simulink model "Fuzzy_and_EKF_STOCAZZO"  (R2021b)
settings: Solver=ode4  StartTime=0.0  StopTime=10.0  FixedStep=1e-2  RelTol=1e-3
values from neighbouring files (symbols this model uses):
  n = length(out.tout)    [Plot_dati.m]
undefined symbols (not defined in the file or in its folder): measure
libraries: fuzblock x1
settings Model: Creator=francescoiotti  LastModifiedBy=pierg
settings ModelReferenceCC: ModelReferenceMinAlgLoopOccurrences=on

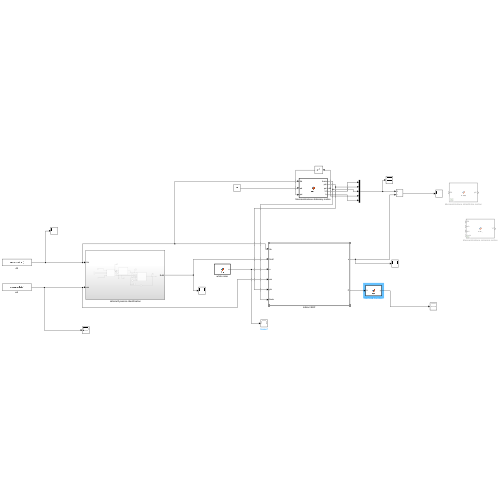
[thumbnail: Simulink's stored preview of the top-level diagram]
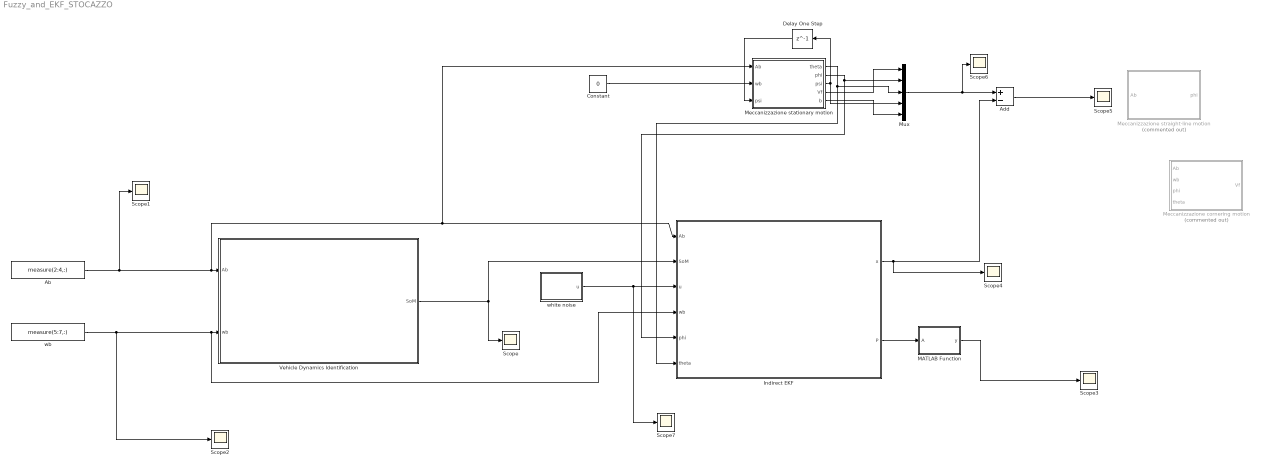
== system Fuzzy_and_EKF_STOCAZZO ==
  Ab : Constant  Value=measure(2:4,:)
  Add : Sum  Inputs=+-
  Constant : Constant  Value=0
  Delay One Step : Delay  DelayLength=1
  Indirect EKF : Subsystem
  MATLAB Function : MATLAB Function  TreatAsAtomicUnit=on
  Meccanizzazione cornering motion : MATLAB Function  Commented=on  TreatAsAtomicUnit=on
  Meccanizzazione stationary motion : MATLAB Function  TreatAsAtomicUnit=on
  Meccanizzazione straight-line motion : MATLAB Function  Commented=on  TreatAsAtomicUnit=on
  Mux : Mux  Inputs=5
  Scope{,1..7} (8 alike) : Scope
  Vehicle Dynamics Identification : Subsystem
  wb : Constant  Value=measure(5:7,:)
  white noise : MATLAB Function  TreatAsAtomicUnit=on
  wires:
  Vehicle Dynamics Identification/1(SoM) -> Indirect EKF/2(SoM), Scope/1
  Ab/1 -> Indirect EKF/1(Ab), Meccanizzazione stationary motion/1(Ab), Vehicle Dynamics Identification/1(Ab), Scope1/1
  wb/1 -> Indirect EKF/4(wb), Vehicle Dynamics Identification/2(wb), Scope2/1
  Indirect EKF/1(x) -> Scope4/1, Add/2
  Indirect EKF/2(P) -> MATLAB Function/1(A)
  Meccanizzazione stationary motion/1(theta) -> Indirect EKF/6(theta), Mux/3
  Meccanizzazione stationary motion/2(phi) -> Indirect EKF/5(phi), Mux/2
  Meccanizzazione stationary motion/3(psi) -> Mux/4, Delay One Step/1
  Delay One Step/1 -> Meccanizzazione stationary motion/3("psi ")
  Meccanizzazione stationary motion/4(Vf) -> Mux/1
  Meccanizzazione stationary motion/5(b) -> Mux/5
  Mux/1 -> Scope6/1, Add/1
  Add/1 -> Scope5/1
  white noise/1(u) -> Indirect EKF/3(u), Scope7/1
  Constant/1 -> Meccanizzazione stationary motion/2(wb)
  MATLAB Function/1(y) -> Scope3/1

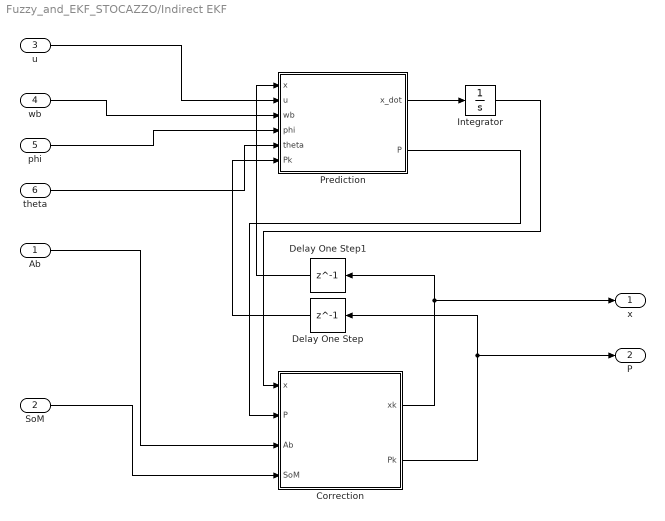
== system Fuzzy_and_EKF_STOCAZZO/Indirect EKF ==
  Ab : Inport
  SoM : Inport  Port=2
  u : Inport  Port=3
  wb : Inport  Port=4
  phi : Inport  Port=5
  theta : Inport  Port=6
  Correction : MATLAB Function  TreatAsAtomicUnit=on
  Delay One Step : Delay  DelayLength=1
  Delay One Step1 : Delay  DelayLength=1
  Integrator : Integrator  InitialCondition=[0 0 0 0 0]'
  Prediction : MATLAB Function  InitFcn=Pk = eye(5)  TreatAsAtomicUnit=on
  x : Outport
  P : Outport  Port=2
  wires:
  Prediction/1(x_dot) -> Integrator/1
  Integrator/1 -> Correction/1(x)
  Ab/1 -> Correction/3(Ab)
  SoM/1 -> Correction/4(SoM)
  Correction/1(xk) -> Delay One Step1/1, x/1
  Correction/2(Pk) -> Delay One Step/1, P/1
  u/1 -> Prediction/2(u)
  Prediction/2(P) -> Correction/2(P)
  wb/1 -> Prediction/3(wb)
  phi/1 -> Prediction/4(phi)
  theta/1 -> Prediction/5(theta)
  Delay One Step/1 -> Prediction/6(Pk)
  Delay One Step1/1 -> Prediction/1(x)

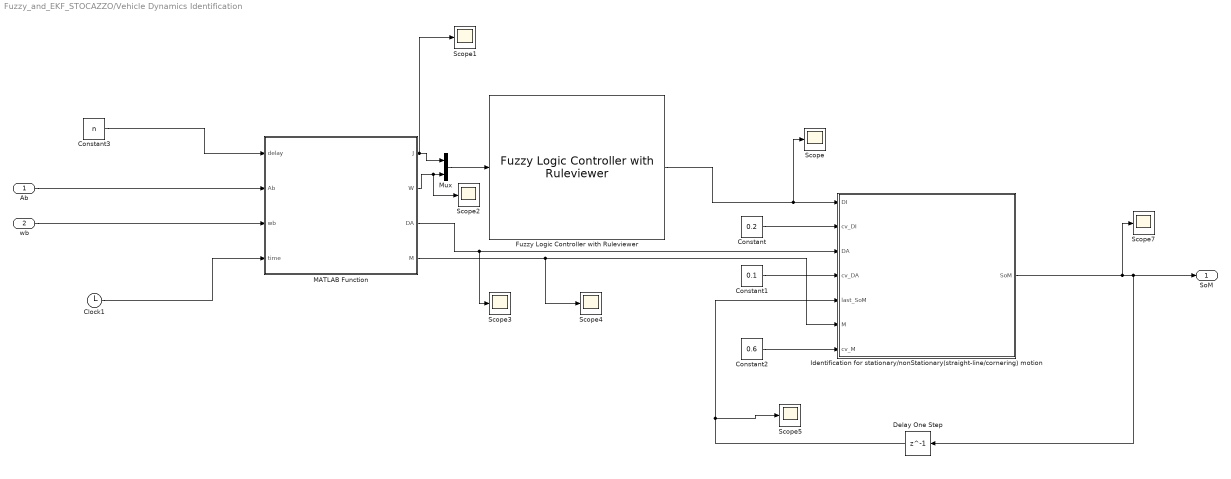
== system Fuzzy_and_EKF_STOCAZZO/Vehicle Dynamics Identification ==
  Ab : Inport
  wb : Inport  Port=2
  Clock1 : Clock
  Constant : Constant  Value=0.2
  Constant1 : Constant  Value=0.1
  Constant2 : Constant  Value=0.6
  Constant3 : Constant  Value=n
  Delay One Step : Delay  DelayLength=1  InitialCondition=1
  Fuzzy Logic Controller with Ruleviewer : fuzblock/Fuzzy Logic  Controller  with Ruleviewer  fismatrix=pippo  Ts=5
  Identification for stationary/nonStationary(straight-line/cornering) motion : MATLAB Function  TreatAsAtomicUnit=on
  MATLAB Function : MATLAB Function  TreatAsAtomicUnit=on
  Mux : Mux  Inputs=2
  Scope{,1..5,7} (7 alike) : Scope
  SoM : Outport
  wires:
  Constant1/1 -> Identification for stationary/nonStationary(straight-line/cornering) motion/4(cv_DA)
  MATLAB Function/3(DA) -> Scope3/1, Identification for stationary/nonStationary(straight-line/cornering) motion/3(DA)
  MATLAB Function/1(J) -> Scope1/1, Mux/1
  Fuzzy Logic Controller with Ruleviewer/1 -> Scope/1, Identification for stationary/nonStationary(straight-line/cornering) motion/1(DI)
  MATLAB Function/4(M) -> Scope4/1, Identification for stationary/nonStationary(straight-line/cornering) motion/6(M)
  Identification for stationary/nonStationary(straight-line/cornering) motion/1(SoM) -> Scope7/1, SoM/1, Delay One Step/1
  Constant2/1 -> Identification for stationary/nonStationary(straight-line/cornering) motion/7(cv_M)
  Constant/1 -> Identification for stationary/nonStationary(straight-line/cornering) motion/2(cv_DI)
  MATLAB Function/2(W) -> Scope2/1, Mux/2
  Mux/1 -> Fuzzy Logic Controller with Ruleviewer/1
  Clock1/1 -> MATLAB Function/4(time)
  wb/1 -> MATLAB Function/3(wb)
  Ab/1 -> MATLAB Function/2(Ab)
  Constant3/1 -> MATLAB Function/1(delay)
  Delay One Step/1 -> Scope5/1, Identification for stationary/nonStationary(straight-line/cornering) motion/5(last_SoM)

== matlab function Fuzzy_and_EKF_STOCAZZO/MATLAB Function ==
  data: A input; y output
function y = fcn(A)
y = norm(A);

== matlab function Fuzzy_and_EKF_STOCAZZO/Meccanizzazione straight-line motion ==
  data: Ab input; phi output
function phi  = mecc(Ab)
% Estraggo le componenti di accelerazione
Abx = Ab(1);
Aby = Ab(2);

% Estraggo le componenti di velocità angolare
% wbx = wb(1);
% wby = wb(2);
% wbz = wb(3);

% Costante
g = 9.81;

% Meccanizzazione
phi = asin(-Aby / sqrt(g^2 - Abx^2));

== matlab function Fuzzy_and_EKF_STOCAZZO/Meccanizzazione stationary motion ==
  data: Ab input; theta output; wb input; psi input; phi output; psi output; Vf output; b output
function [theta, phi, psi, Vf, b] = mecc(Ab, wb, psi)
% Estraggo le componenti di accelerazione
Abx = Ab(1);
Aby = Ab(2);

% Estraggo le componenti di velocità angolare
% wbx = wb(1);
% wby = wb(2);
% wbz = wb(3);

% Costante
g = 9.81;

% Meccanizzazione
theta = asin(Abx/g);
phi = asin(-Aby / sqrt(g^2 - Abx^2));
psi = psi;
Vf = 0;
b = wb;

== matlab function Fuzzy_and_EKF_STOCAZZO/Vehicle Dynamics Identification/Identification for stationary//nonStationary(straight-line//cornering) motion ==
  data: DI input; cv_DI input; DA input; cv_DA input; last_SoM input; M input; SoM output; cv_M input
function SoM = type_of_motion_decision_loop(DI, cv_DI, DA, cv_DA, last_SoM, M, cv_M)

    %% Identification for stationary/nonStationary(straight-line/cornering) motion
    % SoM : state of motion for landend vehicle
    % last_SoM: previous state of motion for landend vehicle
    % 0 := Stationary
    % 1 := straight-line motion
    % 2 := cornering motion
    % notStationary: if 1 the vehicle is not stationary

    notStationary = 1;
    SoM = 0;

    if last_SoM == 0 && DA > cv_DA      
        notStationary = 1;
    elseif	last_SoM && DA < cv_DA && DI < cv_DI
        SoM = 0;
        notStationary = 0;
    else 
        SoM = last_SoM;
        notStationary = 0;
    end
    
    %Run this only if notStactionary
    if notStationary && M > cv_M
        SoM = 2;
    elseif	notStationary && M < cv_M
        SoM = 1;
    elseif notStationary 
        SoM = last_SoM;
    end

    notStationary

== matlab function Fuzzy_and_EKF_STOCAZZO/Vehicle Dynamics Identification/MATLAB Function ==
  data: delay input; Ab input; J output; wb input; time input; W output; DA output; M output
function [J, W, DA, M] = functional_computation(delay, Ab, wb, time)
% Trasformo i tempi in passi
n = int64(delay/1e-2);
t = int64(time/1e-2);
p = int64(1/30/1e-2);
m = n;
% Inizializzo i funzionali
J = 0;
W = 0;
DA = 0;
Mwbz = 0;

% Calcolo J
for i=t-n:t
%   Controllo nel caso in cui t < n ed escludo i termini con indici
%   negativi
    if i > 1
        J = J + abs( norm(Ab(:,i)) - norm(Ab(:,i-1)) );
    end
end

% Calcolo W
for i=t-n:t
%   Controllo nel caso in cui t < n ed escludo i termini con indici
%   negativi
    if i > 1
        W = W + abs( sqrt(wb(1,i)^2 + wb(2,i)^2) ) / double(n);
    end
end


% Calcolo DA
for i=t-p:t
%   Controllo nel caso in cui t < n ed escludo i termini con indici
%   negativi
    if i > 1 && t-p > 0
        DA = DA + abs( Ab(1,i) - Ab(1,t-p) );
    end
end


% Calcolo M
for i=t-m:t
%   Controllo nel caso in cui t < n ed escludo i termini con indici
%   negativi
    if i > 1
        Mwbz = Mwbz + wb(3,i);
    end
end
M = Mwbz / m;

== matlab function Fuzzy_and_EKF_STOCAZZO/Meccanizzazione cornering motion ==
  data: Ab input; wb input; phi input; Vf output; theta input
function Vf  = mecc(Ab, wb, phi, theta)
% Estraggo le componenti di accelerazione
%Abx = Ab(1);
Aby = Ab(2);

% Estraggo le componenti di velocità angolare
% wbx = wb(1);
% wby = wb(2);
wbz = wb(3);

% Costante
g = 9.81;

% Meccanizzazione
Vf = (Aby + g*sin(phi)*cos(theta)) / wbz;

== matlab function Fuzzy_and_EKF_STOCAZZO/Indirect EKF/Prediction ==
  data: x_dot output; x input; u input; wb input; phi input; theta input; Pk input; P output
function [x_dot, P] = prediction(x, u, wb, phi, theta, Pk)

% Estraggo le componenti di velocità angolare
wbx = wb(1);
wby = wb(2);
wbz = wb(3);

% Costante
g = 9.81;

% Definisco gli elementi della matrice F
f13 = -g*cos(theta);
f22 = cos(phi)*tan(theta)*wby - sin(phi)*tan(theta)*wbz;
f23 = sin(phi)*wby/cos(theta)^2 + cos(phi)*wbz/cos(theta)^2;
f32 = -sin(phi)*wby - cos(phi)*wbz;
f42 = cos(phi)*wby/cos(theta) - sin(phi)*wbz/cos(theta);
f43 = sin(phi)*tan(theta)*wby/cos(theta) + cos(phi)*tan(theta)*wbz/cos(theta);

F = [0  0  f13  0  1;
     0 f22 f23  0  0;
     0 f32  0   0  0;
     0 f42 f43  0  0;
     0  0   0   0  0;];

% Definisco gli elementi della matrice G
g23 = sin(phi)*tan(theta);
g24 = cos(phi)*tan(theta);
g33 = cos(phi);
g34 = -sin(phi);
g43 = sin(phi)/cos(theta);
g44 = cos(phi)/cos(theta);

G = [1  0  0   0  0;
     0  1 g23 g24 0;
     0  0 g33 g34 0;
     0  0 g43 g44 0;
     0  0  0   0  1;];

% Formula di predizione dello stato
x_dot = F*x + G*u;


% Definisco la matrice di covarianza del rumore di processo Q
qAbx = 0.001; % densità spettrale
qwbx = 0.1;
qwby = 0.1;
qwbz = 0.1;
qb = 0;
Q = diag([qAbx, qwbx, qwby, qwbz, qb]);

% Formula di predizione della covarianza
P = F*Pk*F' + Q;

== matlab function Fuzzy_and_EKF_STOCAZZO/Indirect EKF/Correction ==
  data: x input; xk output; P input; Ab input; Pk output; SoM input
function [xk, Pk] = correction(x, P, Ab, SoM)
% Estraggo le componenti di accelerazione
Abx = Ab(1);
Aby = Ab(2);
Abz = Ab(3);

% Costante
g = 9.81;

% z = [ Vf ; phi-phi_a ; theta-theta_a ; psi-psi_p ]
if SoM == 0

    % Definisco la matrice H
    H = [ 1 0 0 0 0;
          0 1 0 0 0;
          0 0 1 0 0;
          0 0 0 1 0;];

    % Creo il vettore di rumore   
%     v = [vVf vphi vtheta vpsi]';
     
    % z = [ Vf - 0; phi - phi_a; theta - theta_a; psi - psi_p ]

    % Deviazioni standard rumori di misura in fase stazionaria
    sigma_deltaVf_ZUPT = 0.02;
    sigma_deltaPhi = 0.2;
    sigma_deltaTheta = 0.2;
    sigma_deltaPsi = 0.02;
    % Matrice di covarianza
    R = diag([sigma_deltaVf_ZUPT^2, sigma_deltaPhi^2, sigma_deltaTheta^2, sigma_deltaPsi^2]);

elseif SoM == 1

    % Definisco la matrice H
    H = [ 0 1 0 0 0;];

    % Creo il vettore di rumore
%     v = vphi;
 
    % z = [ phi - phi_a ]

    % Deviazioni standard rumori di misura in fase di movimento lineare
    sigma_deltaPhi = 0.2;
    % Matrice di covarianza
    R = sigma_deltaPhi^2;


elseif SoM == 2

    % Definisco la matrice H
    H = [ 1 0 0 0 0;];

    % Creo il vettore di rumore
%     v = vVf;

    % z = [ Vf - Vf_c ]

    % Deviazioni standard rumori di misura in fase di cornering
    sigma_deltaVf_C = 0.02;
    % Matrice di covarianza
    R = sigma_deltaVf_C^2;

else
%   Caso unaided
    H = zeros(4,5);
    R = eye(4);
    fprintf('Errore su SoM');

end

% Innovazione
z = H * x;
% Covarianza dell'innovazione
S = H * P * H' + R;
L = P * H' * S^(-1);
% Correzione
xk = x + L*z;
% Pk = P - L*S*L';
Pk = (eye(5) - L*H) * P * (eye(5) - L*H)' + L*R*L';

== matlab function Fuzzy_and_EKF_STOCAZZO/white noise ==
  data: u output
function u = fcn()
% Accelerometer 
stdv_a = 0.0055; % standard deviation
Wna = stdv_a*randn(1,1); % White Noise
% Gyroscope
stdv_g = 0.6325; % standard deviation
Wng = stdv_g*randn(1,3); % White Noise

u = [Wna, Wng, 0]';
